simulink model "rotations_test"  (R2018b)
settings: Solver=VariableStepAuto  StartTime=0.0  StopTime=10.0  RelTol=1e-3
values from neighbouring files (symbols this model uses):
  utc_sec = 962131820    [teme2eci_test_init.m]
libraries: time_Lib x1
settings Model: Creator=Kate  LastModifiedBy=taylorreynolds

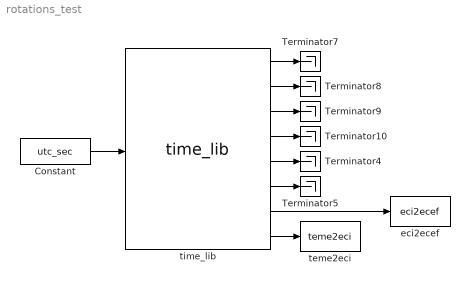
== system rotations_test ==
  Constant : Constant  Value=utc_sec
  Terminator{4..5,7..10} (6 alike) : Terminator
  eci2ecef : ToWorkspace  VariableName=eci2ecef  SaveFormat=Structure With Time  SampleTime=-1
      settings: Save2DSignal=2-D array (concatenate along first dimension)
  teme2eci : ToWorkspace  VariableName=teme2eci  SaveFormat=Structure With Time  SampleTime=-1
      settings: Save2DSignal=2-D array (concatenate along first dimension)
  "time_lib " : time_Lib/time_lib    SystemSampleTime=-1
  wires:
  "time_lib "/7 -> eci2ecef/1
  "time_lib "/6 -> Terminator5/1
  "time_lib "/5 -> Terminator4/1
  "time_lib "/4 -> Terminator10/1
  "time_lib "/3 -> Terminator9/1
  "time_lib "/2 -> Terminator8/1
  "time_lib "/1 -> Terminator7/1
  Constant/1 -> "time_lib "/1
  "time_lib "/8 -> teme2eci/1
